simulink model "lb2"  (R2023b)
settings: Solver=VariableStepAuto  StartTime=0.0  StopTime=10.0  RelTol=1e-3
values from neighbouring files (symbols this model uses):
  H = acker(A, B, des_poles)    [lw2_1.m]
  x0 = [1; 0; 0; 0]    [lw2_2.m]
undefined symbols (not defined in the file or in its folder): A, B, G
settings Model: Creator=kek  LastModifiedBy=kek

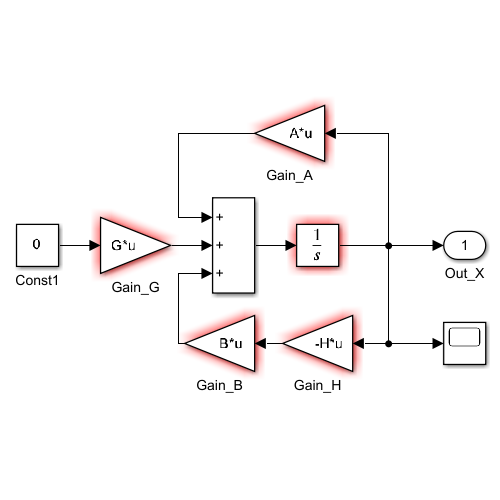
[thumbnail: Simulink's stored preview of the top-level diagram]
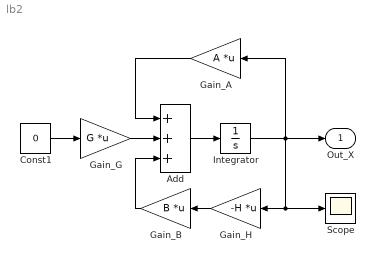
== system lb2 ==
  Add : Sum  Inputs=+++
  Const1 : Constant  Value=0
  Gain_A : Gain  Gain=A  Multiplication=Matrix(K*u)
  Gain_B : Gain  Gain=B  Multiplication=Matrix(K*u)
  Gain_G : Gain  Gain=G  Multiplication=Matrix(K*u)
  Gain_H : Gain  Gain=-H  Multiplication=Matrix(K*u)
  Integrator : Integrator  InitialCondition=x0
  Scope : Scope
  Out_X : Outport
  wires:
  Integrator/1 -> Gain_A/1, Out_X/1, Scope/1, Gain_H/1
  Add/1 -> Integrator/1
  Const1/1 -> Gain_G/1
  Gain_G/1 -> Add/2
  Gain_H/1 -> Gain_B/1
  Gain_A/1 -> Add/1
  Gain_B/1 -> Add/3
